simulink model "IEEE_9bus_new_o"  (R2024a)
settings: Solver=ode45  StartTime=0.0  StopTime=60/60  RelTol=1e-3  EnableMultiTasking=on
PreLoadFcn:
  | faultType = "ABCG";
  | faultLineStr = "Line 7-8";
  | faultDistance = 50;
  | L78_Length = 50;
  | L89_Length = 50;
  | L96_Length = 50;
  | L64_Length = 50;
  | L45_Length = 50;
  | L57_Length = 50;
  | 
  | mdl = load('lineIdentificationModel.mat');
  | lineMdl = mdl.treeModel;
  | 
  | mdl = load('typeIdentificationModelV2.mat');
  | typeMdl = mdl.treeModel;
  | 
  | mdl = load('faultLocationModel.mat');
  | locationMdl = mdl.treeModel;
libraries: dspstat3 x36, simulink x24, spsThreePhasePISectionLineLib x12, spsThreePhaseVIMeasurementLib x12, spsLoadFlowBusLib x9, spsThreePhaseFaultLib x6, jailib x3, spsThreePhaseSourceLib x3, spsThreePhaseTransformerTwoWindingsLib x3, statsLibrary x3, spsThreePhaseBreakerLib x3, sps_lib x1
(part 3 of 3)

== system IEEE_9bus_new_o/Fault Detection/BUS Fault Detection6/Variance Threshold Computation ==
  Var : Inport
  Add Constant : Bias  Bias=-0.03  SaturateOnIntegerOverflow=off
  Clock : Clock
  Constant : Constant  Value=1/60
  Memory : Memory
  Relational Operator1 : RelationalOperator  Operator=<=  OutDataTypeStr=boolean  RndMeth=Simplest  InputSameDT=off
  Switch : Switch  Criteria=u2 > Threshold  SaturateOnIntegerOverflow=off  InputSameDT=off
  ThreshVar : Outport
  wires:
  Add Constant/1 -> ThreshVar/1  "Threshold var"
  Var/1 -> Switch/1
  Constant/1 -> Relational Operator1/2
  Relational Operator1/1 -> Switch/2
  Clock/1 -> Relational Operator1/1
  Switch/1 -> Memory/1, Add Constant/1  "BaseVar"
  Memory/1 -> Switch/3
